simulink model "MKC_H9"  (R2025a)
settings: Solver=VariableStepAuto  StartTime=0.0  StopTime=30  MaxStep=2/50  RelTol=1e-3
settings Model: Creator=Szalay  LastModifiedBy=Szalay

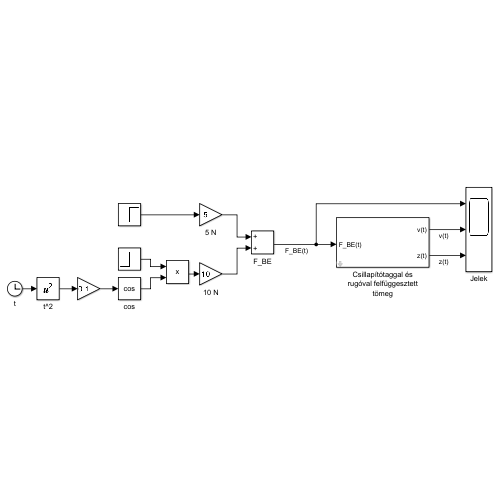
[thumbnail: Simulink's stored preview of the top-level diagram]
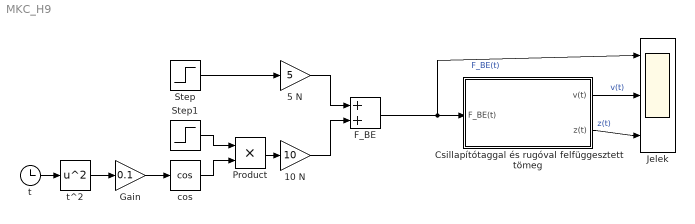
== system MKC_H9 ==
  10 N : Gain  Gain=10
  5 N : Gain  Gain=5
  Csillapítótaggal és rugóval felfüggesztett tömeg : Subsystem  mask(Felfüggesztett rezgő tömeg){tau=2, xi=0.5, c=2, v_0=-0.2, z_0=-0.1}
      mask prompts: tau "Időállandó (s)"; xi "Csillapítási tényező"; c "Rugómerevség (N/m)"; v_0 "Kezdeti sebesség (m/s)"; z_0 "Kezdeti elmozdulás (m)"
      mask help: Csillapítótaggal és rugóval felfüggesztett tömeg.
      mask DialogControl ParameterGroupVar Prompt: Ismert jellemzők
      mask DialogControl Container3 Prompt: Kezdeti értékek
  F_BE : Sum
  Gain : Gain  Gain=0.1
  Jelek : Scope  NumInputPorts=3
      settings: ActiveDisplayYMinimum=-53.197495279178447  ActiveDisplayYMaximum=22.563537212639297
  Product : Product
  Step : Step  Time=10  SampleTime=0
  Step1 : Step  Time=20  SampleTime=0
  cos : Trigonometry  Operator=cos
  t : Clock
  t^2 : Math  Operator=square
  wires:
  F_BE/1 -> Jelek/1, Csillapítótaggal és rugóval felfüggesztett tömeg/1(F_BE(t))  "F_BE(t)"
  Step/1 -> 5 N/1
  5 N/1 -> F_BE/1
  Step1/1 -> Product/1
  cos/1 -> Product/2
  Product/1 -> 10 N/1
  10 N/1 -> F_BE/2
  Gain/1 -> cos/1
  t/1 -> t^2/1
  t^2/1 -> Gain/1
  Csillapítótaggal és rugóval felfüggesztett tömeg/1(v(t)) -> Jelek/2  "v(t)"
  Csillapítótaggal és rugóval felfüggesztett tömeg/2(z(t)) -> Jelek/3  "z(t)"

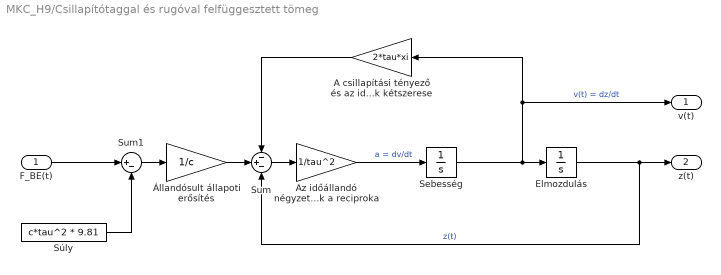
== system MKC_H9/Csillapítótaggal és rugóval felfüggesztett tömeg ==
  F_BE(t) : Inport
  A csillapítási tényező és az időállandó szorzatának kétszerese : Gain  Gain=2*tau*xi
  Az időállandó négyzetének a reciproka : Gain  Gain=1/tau^2
  Elmozdulás : Integrator  InitialCondition=z_0
  Sebesség : Integrator  InitialCondition=v_0
  Sum : Sum  Inputs=-+-
  Sum1 : Sum  Inputs=|+-
  Súly : Constant  Value=c*tau^2 * 9.81
  Állandósult állapoti erősítés : Gain  Gain=1/c
  v(t) : Outport
  z(t) : Outport  Port=2
  wires:
  Sum/1 -> Az időállandó négyzetének a reciproka/1
  Elmozdulás/1 -> z(t)/1, Sum/3  "z(t)"
  A csillapítási tényező és az időállandó szorzatának kétszerese/1 -> Sum/1
  Sebesség/1 -> v(t)/1, A csillapítási tényező és az időállandó szorzatának kétszerese/1, Elmozdulás/1  "v(t) = dz/dt"
  Az időállandó négyzetének a reciproka/1 -> Sebesség/1  "a = dv/dt"
  F_BE(t)/1 -> Sum1/1
  Állandósult állapoti erősítés/1 -> Sum/2
  Súly/1 -> Sum1/2
  Sum1/1 -> Állandósult állapoti erősítés/1
